simulink model "asn5q1"  (R2020b)
settings: Solver=VariableStepAuto  StartTime=0.0  StopTime=30.0  RelTol=1e-3
values from neighbouring files (symbols this model uses):
  g = 9.81    [run_sim_asn5q1.m]    (also in run_sim_asn5q1c.m)
  l1 = 1    [run_sim_asn5q1.m]    (also in run_sim_asn5q1c.m)
  l2 = 1    [run_sim_asn5q1.m]    (also in run_sim_asn5q1c.m)
  m1 = 1    [run_sim_asn5q1.m]    (also in run_sim_asn5q1c.m)
  m2 = 1    [run_sim_asn5q1.m]    (also in run_sim_asn5q1c.m)
  tau = tau_in    [run_sim_asn5q1.m]
  x_0 = x_0_in    [run_sim_asn5q1.m]    (also in run_sim_asn5q1c.m)
settings Model: Creator=zhich  LastModifiedBy=zhich
settings DataIOCC: ExternalInput=x,tau

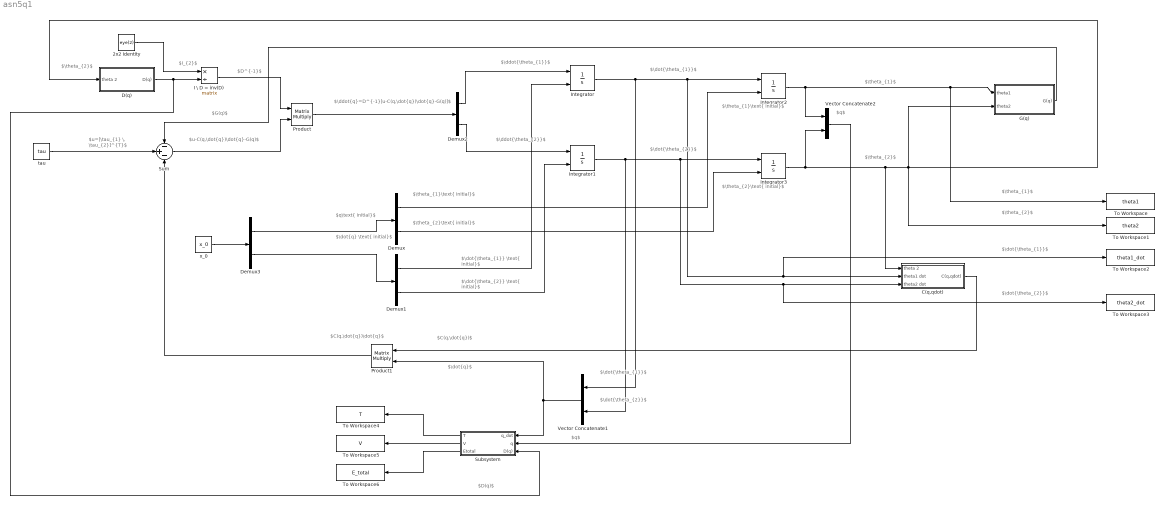
== system asn5q1 ==
  note: $D(q)$
  note: $\ddot{\theta_{1}}$
  note: $\ddot{\theta_{2}}$
  note: $\ddot{q}=D^{-1}[u-C(q,\dot{q})\dot{q}-G(q)]$
  note: $D^{-1}$
  note: $u=[\tau_{1} \, \tau_{2}]^{T}$
  note: $\theta_{1}\text{ initial}$
  note: $\theta_{2}\text{ initial}$
  note: $\dot{\theta_{1}} \text{ initial}$
  note: $\dot{\theta_{2}} \text{ initial}$
  note: $\dot{\theta_{1}}$
  note: $\dot{\theta_{2}}$
  note: $\theta_{1}$
  note: $\theta_{2}$
  note: $\theta_{1}\text{ initial}$
  note: $\theta_{2}\text{ initial}$
  note: $\dot{q}$
  note: $\dot{\theta_{1}}$
  note: $\dot{\theta_{2}}$
  note: $C(q,\dot{q})$
  note: $C(q,\dot{q})\dot{q}$
  note: $u-C(q,\dot{q})\dot{q}-G(q)$
  note: $\theta_{2}$
  note: $I_{2}$
  note: $\theta_{2}$
  note: $\theta_{1}$
  note: $\dot{\theta_{1}}$
  note: $\dot{\theta_{2}}$
  note: $G(q)$
  note: $q$
  note: $q$
  note: $q\text{ initial}$
  note: $\dot{q} \text{ initial}$
  2x2 Identity : Constant  Value=eye(2)
  C(q,qdot) : Subsystem
  D(q) : Subsystem
  Demux{,1..3} (4 alike) : Demux  Outputs=2
  G(q) : Subsystem
  I \ D = inv(D) : Product  Inputs=*/  Multiplication=Matrix(*)
  Integrator{,1..3} (4 alike) : Integrator  InitialConditionSource=external
  Product : Product  Multiplication=Matrix(*)
  Product1 : Product  Multiplication=Matrix(*)
  Subsystem : Subsystem
  Sum : Sum  Inputs=-+-
  To Workspace : ToWorkspace  VariableName=theta1  SaveFormat=Timeseries  SampleTime=-1
  To Workspace1 : ToWorkspace  VariableName=theta2  SaveFormat=Timeseries  SampleTime=-1
  To Workspace2 : ToWorkspace  VariableName=theta1_dot  SaveFormat=Timeseries  SampleTime=-1
  To Workspace3 : ToWorkspace  VariableName=theta2_dot  SaveFormat=Timeseries  SampleTime=-1
  To Workspace4 : ToWorkspace  VariableName=T  SaveFormat=Timeseries  SampleTime=-1
  To Workspace5 : ToWorkspace  VariableName=V  SaveFormat=Timeseries  SampleTime=-1
  To Workspace6 : ToWorkspace  VariableName=E_total  SaveFormat=Timeseries  SampleTime=-1
  Vector Concatenate1 : Concatenate
  Vector Concatenate2 : Concatenate
  tau : Constant  Value=tau
  x_0 : Constant  Value=x_0
  wires:
  D(q)/1(D(q)) -> Subsystem/3(D(q)), I \ D = inv(D)/2
  2x2 Identity/1 -> I \ D = inv(D)/1
  I \ D = inv(D)/1 -> Product/1
  Demux/1 -> Integrator2/2
  Demux/2 -> Integrator3/2
  Sum/1 -> Product/2
  Product/1 -> Demux2/1
  Demux2/1 -> Integrator/1
  Demux2/2 -> Integrator1/1
  Integrator/1 -> To Workspace2/1, C(q,qdot)/2(theta1 dot), Integrator2/1, Vector Concatenate1/1
  Demux1/1 -> Integrator/2
  Demux1/2 -> Integrator1/2
  Integrator1/1 -> To Workspace3/1, C(q,qdot)/3(theta2 dot), Integrator3/1, Vector Concatenate1/2
  Integrator2/1 -> Vector Concatenate2/1, To Workspace/1, G(q)/1(theta1)
  Integrator3/1 -> Vector Concatenate2/2, D(q)/1(theta 2), To Workspace1/1, G(q)/2(theta2), C(q,qdot)/1(theta 2)
  G(q)/1(G(q)) -> Sum/1
  Vector Concatenate1/1 -> Product1/2, Subsystem/1(q_dot)
  C(q,qdot)/1(C(q,qdot)) -> Product1/1
  Product1/1 -> Sum/3
  Vector Concatenate2/1 -> Subsystem/2(q)
  Subsystem/1(T) -> To Workspace4/1
  Subsystem/2(V) -> To Workspace5/1
  Subsystem/3(Etotal) -> To Workspace6/1
  x_0/1 -> Demux3/1
  Demux3/1 -> Demux/1
  Demux3/2 -> Demux1/1
  tau/1 -> Sum/2

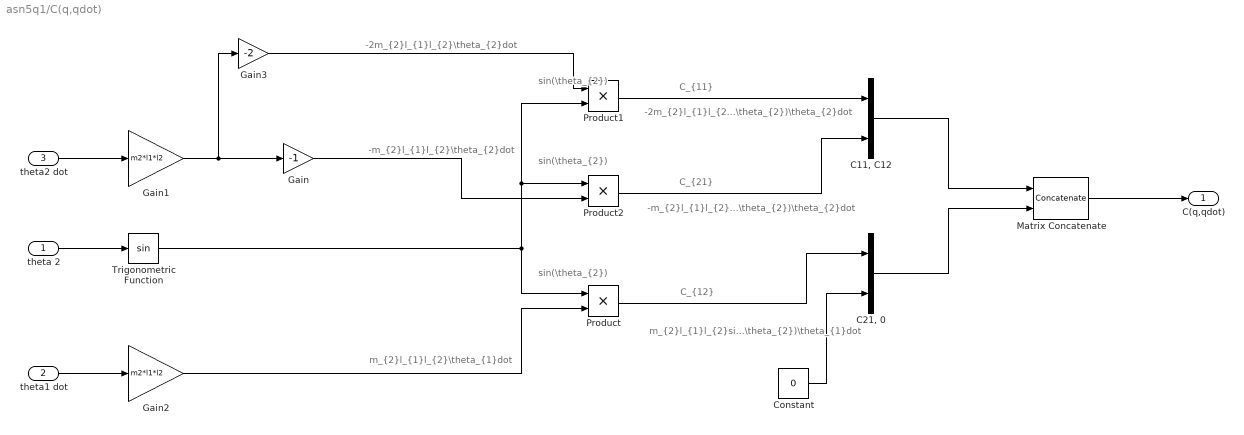
== system asn5q1/C(q,qdot) ==
  note: C_{21}
  note: -m_{2}l_{1}l_{2}\theta_{2}dot
  note: sin(\theta_{2})
  note: sin(\theta_{2})
  note: sin(\theta_{2})
  note: -2m_{2}l_{1}l_{2}\theta_{2}dot
  note: m_{2}l_{1}l_{2}\theta_{1}dot
  note: -m_{2}l_{1}l_{2}sin(\theta_{2})\theta_{2}dot
  note: C_{12}
  note: -2m_{2}l_{1}l_{2}sin(\theta_{2})\theta_{2}dot
  note: m_{2}l_{1}l_{2}sin(\theta_{2})\theta_{1}dot
  note: C_{11}
  theta 2 : Inport
  theta1 dot : Inport  Port=2
  theta2 dot : Inport  Port=3
  "C11, C12" : Concatenate
  "C21, 0" : Concatenate
  Constant : Constant  Value=0
  Gain : Gain  Gain=-1
  Gain1 : Gain  Gain=m2*l1*l2
  Gain2 : Gain  Gain=m2*l1*l2
  Gain3 : Gain  Gain=-2
  Matrix Concatenate : Concatenate  Mode=Multidimensional array  ConcatenateDimension=2
  Product : Product
  Product1 : Product
  Product2 : Product
  Trigonometric Function : Trigonometry
  C(q,qdot) : Outport
  wires:
  theta 2/1 -> Trigonometric Function/1
  theta1 dot/1 -> Gain2/1
  theta2 dot/1 -> Gain1/1
  Gain2/1 -> Product/2
  Trigonometric Function/1 -> Product/1, Product1/2, Product2/1
  Product/1 -> "C21, 0"/1
  Gain1/1 -> Gain3/1, Gain/1
  Gain/1 -> Product2/2
  Gain3/1 -> Product1/1
  Product2/1 -> "C11, C12"/2
  Matrix Concatenate/1 -> C(q,qdot)/1
  Product1/1 -> "C11, C12"/1
  "C11, C12"/1 -> Matrix Concatenate/1
  Constant/1 -> "C21, 0"/2
  "C21, 0"/1 -> Matrix Concatenate/2

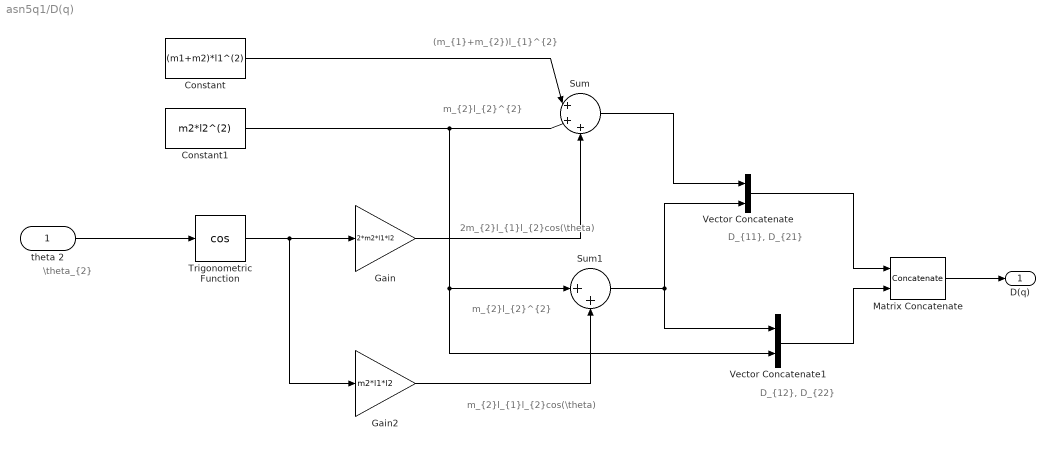
== system asn5q1/D(q) ==
  note: D_{12}, D_{22}
  note: D_{11}, D_{21}
  note: (m_{1}+m_{2})l_{1}^{2}
  note: \theta_{2}
  note: m_{2}l_{2}^{2}
  note: 2m_{2}l_{1}l_{2}cos(\theta)
  note: m_{2}l_{2}^{2}
  note: m_{2}l_{1}l_{2}cos(\theta)
  theta 2 : Inport
  Constant : Constant  Value=(m1+m2)*l1^(2)
  Constant1 : Constant  Value=m2*l2^(2)
  Gain : Gain  Gain=2*m2*l1*l2
  Gain2 : Gain  Gain=m2*l1*l2
  Matrix Concatenate : Concatenate  Mode=Multidimensional array  ConcatenateDimension=2
  Sum : Sum  Inputs=|+++
  Sum1 : Sum  Inputs=|++
  Trigonometric Function : Trigonometry  Operator=cos
  Vector Concatenate : Concatenate
  Vector Concatenate1 : Concatenate
  D(q) : Outport
  wires:
  theta 2/1 -> Trigonometric Function/1
  Trigonometric Function/1 -> Gain/1, Gain2/1
  Vector Concatenate/1 -> Matrix Concatenate/1
  Matrix Concatenate/1 -> D(q)/1
  Sum/1 -> Vector Concatenate/1
  Gain/1 -> Sum/3
  Constant1/1 -> Vector Concatenate1/2, Sum1/1, Sum/2
  Gain2/1 -> Sum1/2
  Sum1/1 -> Vector Concatenate1/1, Vector Concatenate/2
  Constant/1 -> Sum/1
  Vector Concatenate1/1 -> Matrix Concatenate/2

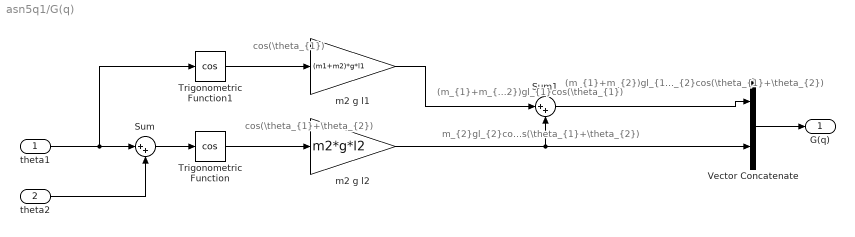
== system asn5q1/G(q) ==
  note: cos(\theta_{1})
  note: (m_{1}+m_{2})gl_{1}cos(\theta_{1})+m_{2}gl_{2}cos(\theta_{1}+\theta_{2})
  note: (m_{1}+m_{2})gl_{1}cos(\theta_{1})
  note: m_{2}gl_{2}cos(\theta_{1}+\theta_{2})
  note: cos(\theta_{1}+\theta_{2})
  theta1 : Inport
  theta2 : Inport  Port=2
  Sum : Sum  Inputs=|++
  Sum1 : Sum  Inputs=|++
  Trigonometric Function : Trigonometry  Operator=cos
  Trigonometric Function1 : Trigonometry  Operator=cos
  Vector Concatenate : Concatenate
  m2 g l1 : Gain  Gain=(m1+m2)*g*l1
  m2 g l2 : Gain  Gain=m2*g*l2
  G(q) : Outport
  wires:
  theta1/1 -> Trigonometric Function1/1, Sum/1
  theta2/1 -> Sum/2
  Sum/1 -> Trigonometric Function/1
  Trigonometric Function/1 -> m2 g l2/1
  Vector Concatenate/1 -> G(q)/1
  m2 g l2/1 -> Sum1/2, Vector Concatenate/2
  Trigonometric Function1/1 -> m2 g l1/1
  m2 g l1/1 -> Sum1/1
  Sum1/1 -> Vector Concatenate/1

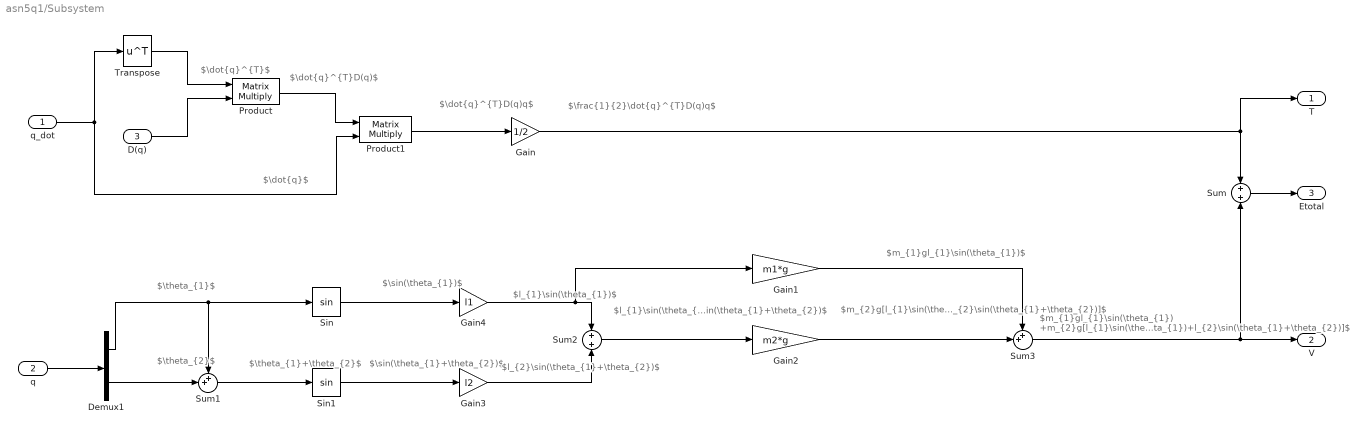
== system asn5q1/Subsystem ==
  note: $\dot{q}^{T}$
  note: $\dot{q}^{T}D(q)$
  note: $\dot{q}$
  note: $\dot{q}^{T}D(q)q$
  note: $\frac{1}{2}\dot{q}^{T}D(q)q$
  note: $\theta_{1}$
  note: $\theta_{2}$
  note: $\theta_{1}+\theta_{2}$
  note: $\sin(\theta_{1}+\theta_{2})$
  note: $\sin(\theta_{1})$
  note: $l_{1}\sin(\theta_{1})$
  note: $l_{2}\sin(\theta_{1}+\theta_{2})$
  note: $l_{1}\sin(\theta_{1})+l_{2}\sin(\theta_{1}+\theta_{2})$
  note: $m_{2}g[l_{1}\sin(\theta_{1})+l_{2}\sin(\theta_{1}+\theta_{2})]$
  note: $m_{1}gl_{1}\sin(\theta_{1})$
  note: $m_{1}gl_{1}\sin(\theta_{1}) +m_{2}g[l_{1}\sin(\theta_{1})+l_{2}\sin(\theta_{1}+\theta_{2})]$
  q_dot : Inport
  q : Inport  Port=2
  D(q) : Inport  Port=3
  Demux1 : Demux  Outputs=2
  Gain : Gain  Gain=1/2
  Gain1 : Gain  Gain=m1*g
  Gain2 : Gain  Gain=m2*g
  Gain3 : Gain  Gain=l2
  Gain4 : Gain  Gain=l1
  Product : Product  Multiplication=Matrix(*)
  Product1 : Product  Multiplication=Matrix(*)
  Sin : Trigonometry
  Sin1 : Trigonometry
  Sum : Sum
  Sum1 : Sum  Inputs=++|
  Sum2 : Sum
  Sum3 : Sum  Inputs=++|
  Transpose : Math  Operator=transpose  SaturateOnIntegerOverflow=on
  T : Outport
  V : Outport  Port=2
  Etotal : Outport  Port=3
  wires:
  q_dot/1 -> Transpose/1, Product1/2
  q/1 -> Demux1/1
  Transpose/1 -> Product/1
  D(q)/1 -> Product/2
  Product/1 -> Product1/1
  Product1/1 -> Gain/1
  Gain/1 -> T/1, Sum/1
  Sum/1 -> Etotal/1
  Demux1/1 -> Sin/1, Sum1/1
  Demux1/2 -> Sum1/2
  Sum1/1 -> Sin1/1
  Sin/1 -> Gain4/1
  Sin1/1 -> Gain3/1
  Gain4/1 -> Gain1/1, Sum2/1
  Gain3/1 -> Sum2/2
  Sum2/1 -> Gain2/1
  Gain2/1 -> Sum3/2
  Gain1/1 -> Sum3/1
  Sum3/1 -> Sum/2, V/1
